simulink model "parte4_eje4_TGOV1"  (R2019b)
settings: Solver=VariableStepAuto  StartTime=0.0  StopTime=10.0  RelTol=1e-3
values from neighbouring files (symbols this model uses):
  R = 0.05    [parte4_eje2_Thidraulica_const.m]
undefined symbols (not defined in the file or in its folder): Dt, H, Kd, T1, T2
settings Model: Creator=cjuar  LastModifiedBy=cjuar

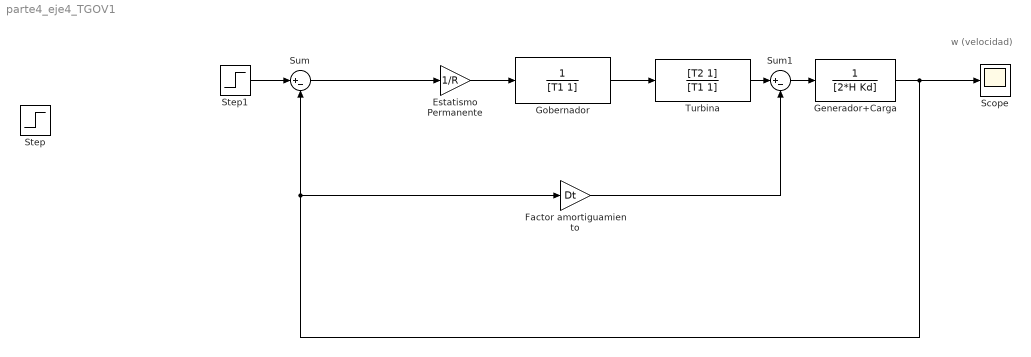
== system parte4_eje4_TGOV1 ==
  note: w (velocidad)
  Estatismo Permanente : Gain  Gain=1/R
  Factor amortiguamiento : Gain  Gain=Dt
  Generador+Carga : TransferFcn  Denominator=[2*H Kd]
  Gobernador : TransferFcn  Denominator=[T1 1]
  Scope : Scope
  Step : Step  SampleTime=0
  Step1 : Step  SampleTime=0
  Sum : Sum  Inputs=|+-
  Sum1 : Sum  Inputs=|+-
  Turbina : TransferFcn  Numerator=[T2 1]  Denominator=[T1 1]
  wires:
  Gobernador/1 -> Turbina/1
  Estatismo Permanente/1 -> Gobernador/1
  Sum/1 -> Estatismo Permanente/1
  Factor amortiguamiento/1 -> Sum1/2
  Turbina/1 -> Sum1/1
  Sum1/1 -> Generador+Carga/1
  Generador+Carga/1 -> Scope/1, Factor amortiguamiento/1, Sum/2
  Step1/1 -> Sum/1
